simulink model "GNSS_pose_conversion"  (R2021a)
settings: configuration reference "AION_IDS_Speedgoat" (kept outside this file)
libraries: simulink x1
settings Model: DataDictionary=GNSS_Pose_Conversion.sldd  Creator=xinrui  LastModifiedBy=Administrator
settings ConfigSetRef: SourceName=AION_IDS_Speedgoat

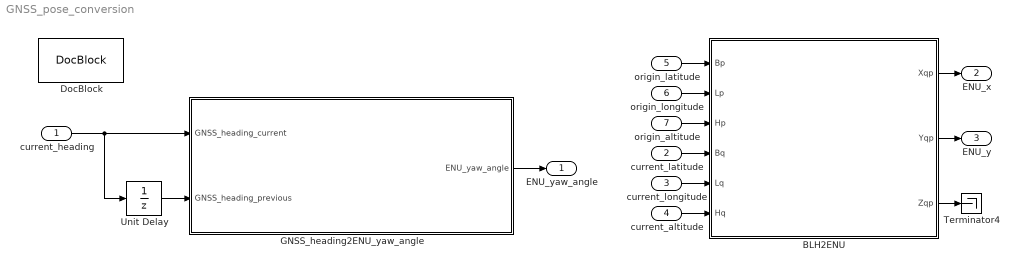
== system GNSS_pose_conversion ==
  current_heading : Inport  OutDataTypeStr=double  PortDimensions=1
  current_latitude : Inport  Port=2  OutDataTypeStr=double  PortDimensions=1
  current_longitude : Inport  Port=3  OutDataTypeStr=double  PortDimensions=1
  current_altitude : Inport  Port=4  OutDataTypeStr=double  PortDimensions=1
  origin_latitude : Inport  Port=5  OutDataTypeStr=double  PortDimensions=1
  origin_longitude : Inport  Port=6  OutDataTypeStr=double  PortDimensions=1
  origin_altitude : Inport  Port=7  OutDataTypeStr=double  PortDimensions=1
  BLH2ENU : Subsystem
  DocBlock : simulink/Model-Wide Utilities/DocBlock  DocumentType=HTML  mask(DocBlock){}
      mask Display:
      | plot([.8 0 0 1 1 .8 .8 1],[1 1 0 0 .8 1 .8 .8]);
      | text(.5,.6,'CHANGELOG','horizontalalignment','center');
      | text(.95,.05,get_param(gcb,'DocumentType'),'verticalalignment','bottom','horizontalalignment','right');
  GNSS_heading2ENU_yaw_angle : MATLAB Function  TreatAsAtomicUnit=on
  Terminator4 : Terminator
  Unit Delay : UnitDelay  SampleTime=-1  HasFrameUpgradeWarning=on
  ENU_yaw_angle : Outport  OutDataTypeStr=double  PortDimensions=1
  ENU_x : Outport  Port=2  OutDataTypeStr=double  PortDimensions=1
  ENU_y : Outport  Port=3  OutDataTypeStr=double  PortDimensions=1
  wires:
  GNSS_heading2ENU_yaw_angle/1(ENU_yaw_angle) -> ENU_yaw_angle/1
  origin_latitude/1 -> BLH2ENU/1(Bp)
  current_heading/1 -> Unit Delay/1, GNSS_heading2ENU_yaw_angle/1(GNSS_heading_current)
  BLH2ENU/3(Zqp) -> Terminator4/1
  origin_altitude/1 -> BLH2ENU/3(Hp)
  BLH2ENU/1(Xqp) -> ENU_x/1
  current_latitude/1 -> BLH2ENU/4(Bq)
  current_longitude/1 -> BLH2ENU/5(Lq)
  BLH2ENU/2(Yqp) -> ENU_y/1
  current_altitude/1 -> BLH2ENU/6(Hq)
  origin_longitude/1 -> BLH2ENU/2(Lp)
  Unit Delay/1 -> GNSS_heading2ENU_yaw_angle/2(GNSS_heading_previous)

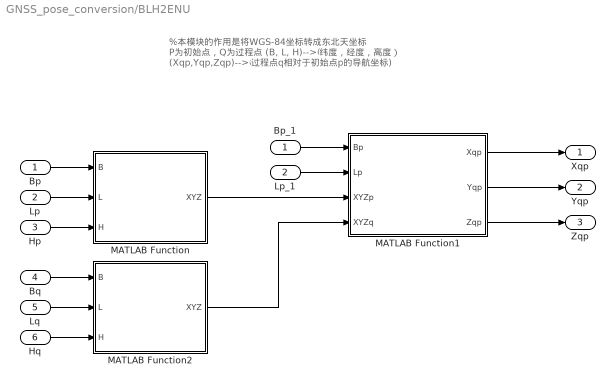
== system GNSS_pose_conversion/BLH2ENU ==
  note: %本模块的作用是将WGS-84坐标转成东北天坐标
      | P为初始点，Q为过程点
      | (B, L, H)-->(纬度，经度，高度）
      | (Xqp,Yqp,Zqp)-->(过程点q相对于初始点p的导航坐标)
  Bp : Inport  OutDataTypeStr=double  PortDimensions=1
  Lp : Inport  Port=2  OutDataTypeStr=double  PortDimensions=1
  Hp : Inport  Port=3  OutDataTypeStr=double  PortDimensions=1
  Bq : Inport  Port=4  OutDataTypeStr=double  PortDimensions=1
  Lq : Inport  Port=5  OutDataTypeStr=double  PortDimensions=1
  Hq : Inport  Port=6  OutDataTypeStr=double  PortDimensions=1
  Bp_1 : InportShadow  OutDataTypeStr=double  PortDimensions=1
  Lp_1 : InportShadow  Port=2  OutDataTypeStr=double  PortDimensions=1
  MATLAB Function : MATLAB Function  TreatAsAtomicUnit=on
  MATLAB Function1 : MATLAB Function  TreatAsAtomicUnit=on
  MATLAB Function2 : MATLAB Function  TreatAsAtomicUnit=on
  Xqp : Outport  OutDataTypeStr=double  PortDimensions=1
  Yqp : Outport  Port=2  OutDataTypeStr=double  PortDimensions=1
  Zqp : Outport  Port=3  OutDataTypeStr=double  PortDimensions=1
  wires:
  MATLAB Function2/1(XYZ) -> MATLAB Function1/4(XYZq)
  Lp_1/1 -> MATLAB Function1/2(Lp)
  Lq/1 -> MATLAB Function2/2(L)
  Bp_1/1 -> MATLAB Function1/1(Bp)
  Hq/1 -> MATLAB Function2/3(H)
  Lp/1 -> MATLAB Function/2(L)
  MATLAB Function/1(XYZ) -> MATLAB Function1/3(XYZp)
  Hp/1 -> MATLAB Function/3(H)
  Bp/1 -> MATLAB Function/1(B)
  Bq/1 -> MATLAB Function2/1(B)
  MATLAB Function1/1(Xqp) -> Xqp/1
  MATLAB Function1/2(Yqp) -> Yqp/1
  MATLAB Function1/3(Zqp) -> Zqp/1

== matlab function GNSS_pose_conversion/BLH2ENU/MATLAB Function ==
  data: B input double size=1; XYZ output double; L input double size=1; H input double size=1
% 本函数将GPS给出的“WGS84坐标系”（纬度， 经度，高度）转换成“地心大地坐标系”（X, Y, Z)
function XYZ = wgs84toxyz(B, L, H)
% WGS-84坐标系使用的地球椭球参数
ADCU1 = 6378137; % 长半轴（m)
b = 6356752.31414; % 短半轴（m）
e = 0.0818191910428; % 偏心率
% 将经度纬度转换成弧度值方便使用三角函数
B = B*pi/180; %纬度转换成弧度
L = L*pi/180; %经度转换成弧度
% 由该点的纬度B计算地球椭球卯酉圈曲率半径Rn
Rn = ADCU1^2/sqrt(ADCU1^2*(cos(B))^2+b^2*(sin(B))^2);
% 计算地心大地坐标X
X = (Rn + H)*cos(B)*cos(L);
% 计算地心大地坐标Y
Y = (Rn + H)*cos(B)*sin(L);
% 计算地心大地坐标Z
Z = (Rn + H-e^2*Rn)*sin(B);
XYZ = [X, Y, Z];

== matlab function GNSS_pose_conversion/GNSS_heading2ENU_yaw_angle ==
  data: GNSS_heading_current input double size=1; ENU_yaw_angle output double size=1; GNSS_heading_previous input double size=1
% 组合惯导航向角转为东北天横摆角
function ENU_yaw_angle = GNSS_heading2ENU_yaw_angle(GNSS_heading_current, GNSS_heading_previous)
%   1.输入参数：
%       (1)GNSS_heading_current     本周期组合惯导航向角，deg
%       (2)GNSS_heading_previous    上周期组合惯导航向角，deg
%   2.输出参数：
%       (1)ENU_yaw_angle            东北天横摆角，deg

%% 静态变量声明
persistent cumulative_counter;       % 累积计数器，用于存储角度转过的圈数，顺时针累积为正，逆时针累积为负

%% 静态变量初始化
if isempty(cumulative_counter)
   cumulative_counter = 0;
end

%% 将0-360度的航向角转换为无上下限的累计角度
delta_angle = GNSS_heading_current - GNSS_heading_previous;

% 变化角度小于-350度，认为是从350多度顺时针转过零点，计数器加1
if -350 > delta_angle
    cumulative_counter = cumulative_counter + 1;
end

% 变化角度大于350度，认为是从0度逆时针转过零点，计数器减1
if 350 < delta_angle
    cumulative_counter = cumulative_counter - 1;
end

%% 角度转换
% 根据计数器累积航向角，用90度减去它转换成东北天横摆角
ENU_yaw_angle = 90 - (GNSS_heading_current + 360 * cumulative_counter);

end

== matlab function GNSS_pose_conversion/BLH2ENU/MATLAB Function1 ==
  data: Bp input double size=1; Lp input double size=1; Xqp output double size=1; XYZp input double; XYZq input double; Yqp output double size=1; Zqp output double size=1
% 本函数将“地心大地坐标系”转换成“局部切平面直角坐标系”（东北天ENU)
% 函数的输入XYZp, XYZq分别为p, q两点的“地心大地坐标”
% P点为初始点（Bp, Lp, Hp)/(Xp, Yp, Zp)，Q点为过程点，则Q点相对于P点的导航坐标为（Xqp, Yqp, Zqp）
function [Xqp, Yqp, Zqp] = xyztoENU(Bp, Lp, XYZp, XYZq)
%% P点的坐标（Bp, Lp, Hp)和(Xp, Yp, Zp)
% 将P点的经纬度转成弧度
Bp = Bp * pi / 180;
Lp = Lp * pi / 180;
%% 建立坐标转换的系数矩阵A
A = zeros(3,3);
A(1, 1) = -sin(Lp);
A(1, 2) = cos(Lp);
A(1, 3) = 0;
A(2, 1) = -sin(Bp)*cos(Lp);
A(2, 2) = -sin(Bp)*sin(Lp);
A(2, 3) = cos(Bp);
A(3, 1) = cos(Bp)*cos(Lp);
A(3, 2) = cos(Bp)*sin(Lp);
A(3, 3) = sin(Bp);
% QP两点的坐标差值dis_qp
dis_qp = XYZq - XYZp;
dis_qp = dis_qp'; % 将坐标转成列向量
% return 结果
result = A*dis_qp;
Xqp= result(1);
Yqp= result(2);
Zqp= result(3);

== matlab function GNSS_pose_conversion/BLH2ENU/MATLAB Function2 ==
  data: B input double size=1; XYZ output double; L input double size=1; H input double size=1
% 本函数将GPS给出的“WGS84坐标系”（纬度， 经度，高度）转换成“地心大地坐标系”（X, Y, Z)
function XYZ = wgs84toxyz(B, L, H)
% WGS-84坐标系使用的地球椭球参数
ADCU1 = 6378137; % 长半轴（m)
b = 6356752.31414; % 短半轴（m）
e = 0.0818191910428; % 偏心率
% 将经度纬度转换成弧度值方便使用三角函数
B = B*pi/180; %纬度转换成弧度
L = L*pi/180; %经度转换成弧度
% 由该点的纬度B计算地球椭球卯酉圈曲率半径Rn
Rn = ADCU1^2/sqrt(ADCU1^2*(cos(B))^2+b^2*(sin(B))^2);
% 计算地心大地坐标X
X = (Rn + H)*cos(B)*cos(L);
% 计算地心大地坐标Y
Y = (Rn + H)*cos(B)*sin(L);
% 计算地心大地坐标Z
Z = (Rn + H-e^2*Rn)*sin(B);
XYZ = [X, Y, Z];
